simulink model "UpDownCounter"  (R2013a)
settings: Solver=ode45  StartTime=0.0  StopTime=10.0  RelTol=1e-3
settings Model: Creator=ajdin  LastModifiedBy=ajdin

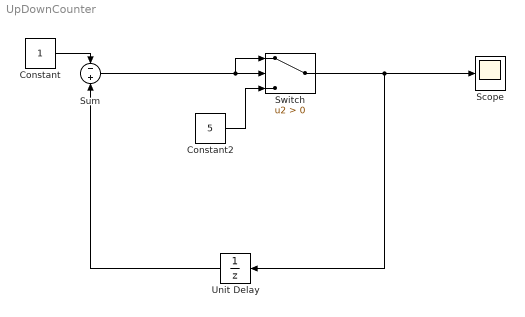
== system UpDownCounter ==
  Constant : Constant
  Constant2 : Constant  Value=5
  Scope : Scope
      settings: YMin=-1  YMax=8
  Sum : Sum  Inputs=-+
  Switch : Switch  Criteria=u2 > Threshold
  Unit Delay : UnitDelay  SampleTime=-1
  wires:
  Constant/1 -> Sum/1
  Unit Delay/1 -> Sum/2
  Sum/1 -> Switch/1, Switch/2
  Constant2/1 -> Switch/3
  Switch/1 -> Scope/1, Unit Delay/1
